simulink model "ProjectGroup5_Simulinkmodell_with_electric_motor_model"  (R2021a)
settings: Solver=FixedStepAuto  StartTime=0.0  StopTime=120  FixedStep=0.001  RelTol=1e-3
model workspace (MATLAB code in the model file):
  | g = 9.81;
  | m = 12600;
  | v = 0.7518;
  | r = 0.2323/2;
  | cd = 1.8;
  | p = 1;
  | A = 1.5;
  | 
  | Fd = 0.5*cd*p*A*v^2;
  | Fb = 1000*9.81*2;
  | E = v*g*m
  | wl = 60*v*4/r
  | Fm = m*g;
  | F = (-Fd-Fm+Fb)/4
  | 
  | T = F*r
undefined symbols (not defined in the file or in its folder): Gf, I_max, I_min, j, k, k2, ki, kp, L_m, L_m_hat, L_r, L_sig, magnitude, n_p, omega_1_N, psi_ref, R_a, R_R, R_R_hat, R_s, T_23, T_32, V_base, v_max
libraries: fl_lib x20, nesl_utility x10, CustomComponents_lib x6, pid_lib x2, sdl_lib x1, simulink x1
settings Model: Creator=simonmarheim  LastModifiedBy=michaerh
settings SolverCC: AlgebraicLoopSolver=TrustRegion
settings DebuggingCC: ArithmeticOperatorsInVariantConditions=warning
settings SFSimCC: CustomCodeUndefinedFunction=UseInterfaceOnly

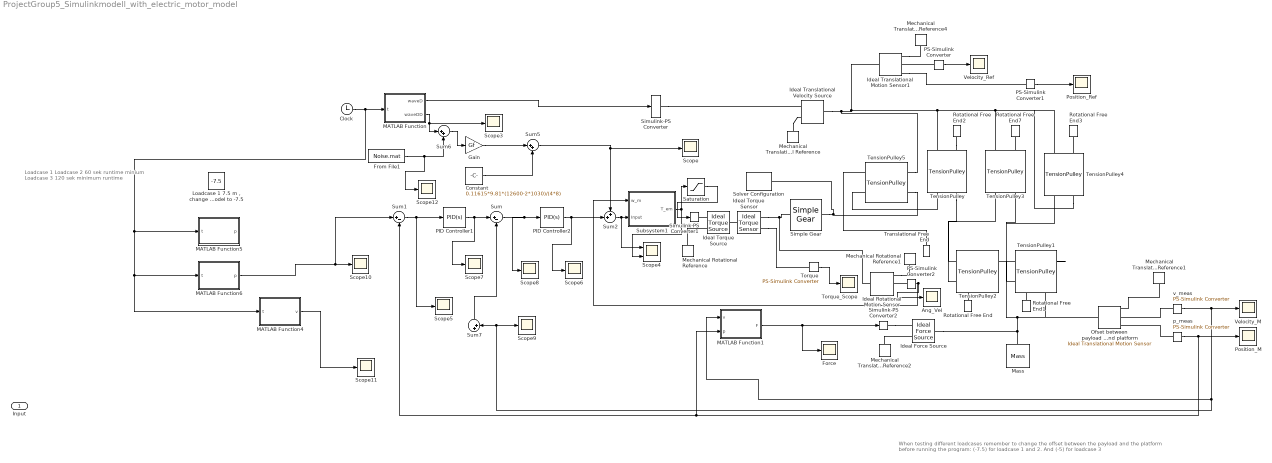
== system ProjectGroup5_Simulinkmodell_with_electric_motor_model ==
  note: Loadcase 1
      |
      | Loadcase 2
      | 60 sek runtime minium
      |
      | Loadcase 3
      | 120 sek minimum runtime
  note: When testing different loadcases remember to change the offset between the payload and the platform before running the program: (-7.5) for loadcase 1 and 2. And (-5) for loadcase 3
  Input : Inport
  Ang_Vel : Scope
  Clock : Clock
      settings: Decimation=25
  Constant : Constant  Value=0.11615*9.81*(12600-2*1030)/(4*8)
  Force : Scope
  From File1 : FromFile  FileName=Noise.mat  SampleTime=0.001
  Gain : Gain  Gain=Gf
  Ideal Force Source : fl_lib/Mechanical/Mechanical Sources/Ideal Force Source
  Ideal Rotational Motion Sensor : fl_lib/Mechanical/Mechanical Sensors/Ideal Rotational Motion Sensor  wrap_angle=simscape.enum.onoff.off  offset=0 rad
  Ideal Torque Sensor : fl_lib/Mechanical/Mechanical Sensors/Ideal Torque Sensor
  Ideal Torque Source : fl_lib/Mechanical/Mechanical Sources/Ideal Torque Source
  Ideal Translational Motion Sensor1 : fl_lib/Mechanical/Mechanical Sensors/Ideal Translational Motion Sensor  offset=0 m
  Ideal Translational Velocity Source : fl_lib/Mechanical/Mechanical Sources/Ideal Translational Velocity Source
  "Loadcase 1 7.5 m , change setpoint in model to -7.5" : Constant  Value=-7.5
  MATLAB Function : MATLAB Function  TreatAsAtomicUnit=on
  MATLAB Function1 : MATLAB Function  TreatAsAtomicUnit=on
  MATLAB Function4 : MATLAB Function  TreatAsAtomicUnit=on
  MATLAB Function5 : MATLAB Function  TreatAsAtomicUnit=on
  MATLAB Function6 : MATLAB Function  TreatAsAtomicUnit=on
  Mass : fl_lib/Mechanical/Translational Elements/Mass  mass=12600 kg  num_ports=foundation.enum.numPorts2.one  v_specify=off  v_priority=High  v=0 m/s  v_nominal_specify=off  v_nominal_unit=m/s  v_nominal_value=1  f_specify=off  f_priority=None  f=0 N  f_nominal_specify=off  f_nominal_unit=N  f_nominal_value=1
  Mechanical Rotational Reference : fl_lib/Mechanical/Rotational Elements/Mechanical Rotational Reference
  Mechanical Rotational Reference1 : fl_lib/Mechanical/Rotational Elements/Mechanical Rotational Reference
  Mechanical Translational Reference{,1..2,4} (4 alike) : fl_lib/Mechanical/Translational Elements/Mechanical Translational Reference
  Ofset between payload and platform : fl_lib/Mechanical/Mechanical Sensors/Ideal Translational Motion Sensor  offset=-5 m
  PID Controller1 : pid_lib/PID Controller  Controller=PID  Form=Parallel  TimeDomain=Continuous-time  UseExternalTs=off  SampleTime=-1  IntegratorMethod=Forward Euler  FilterMethod=Forward Euler  ControllerParametersSource=internal  P=950  I=100  D=0  UseFilter=on  N=100  TunerSelectOption=Transfer Function Based (PID Tuner App)  InitialConditionSource=internal  InitialConditionForIntegrator=0  InitialConditionForFilter=0  DifferentiatorICPrevScaledInput=0  ExternalReset=none  TrackingMode=off  Kt=1  LimitOutput=off  SatLimitsSource=internal  UpperSaturationLimit=inf  LowerSaturationLimit=-inf  LinearizeAsGain=on  AntiWindupMode=none  Kb=1  POutMin=[]  POutMax=[]  IOutMin=[]  IOutMax=[]  DOutMin=[]  DOutMax=[]  NOutMin=[]  NOutMax=[]  SumOutMin=[]  SumOutMax=[]  SaturationOutMin=[]  SaturationOutMax=[]  PParamMin=[]  PParamMax=[]  IParamMin=[]  IParamMax=[]  DParamMin=[]  DParamMax=[]  NParamMin=[]  NParamMax=[]  KbParamMin=[]  KbParamMax=[]  KtParamMin=[]  KtParamMax=[]  KbOutMin=[]  KbOutMax=[]  KtOutMin=[]  KtOutMax=[]  IntegratorOutMin=[]  IntegratorOutMax=[]  FilterOutMin=[]  FilterOutMax=[]  SumI1OutMin=[]  SumI1OutMax=[]  SumI2OutMin=[]  SumI2OutMax=[]  SumI3OutMin=[]  SumI3OutMax=[]  SumI4OutMin=[]  SumI4OutMax=[]  SumDOutMin=[]  SumDOutMax=[]  DifferentiatorOutMin=[]  DifferentiatorOutMax=[]  FilterDiffOutCoefMin=[]  FilterDiffOutCoefMax=[]  ReciprocalOutMin=[]  ReciprocalOutMax=[]  SumDenOutMin=[]  SumDenOutMax=[]  SumNumOutMin=[]  SumNumOutMax=[]  DivideOutMin=[]  DivideOutMax=[]  UdiffTsProdOutMin=[]  UdiffTsProdOutMax=[]  NTsProdOutMin=[]  NTsProdOutMax=[]  UintegralTsProdOutMin=[]  UintegralTsProdOutMax=[]  UngainTsProdOutMin=[]  UngainTsProdOutMax=[]  IntegratorContinuousStateAttributes=''  IntegratorStateMustResolveToSignalObject=off  IntegratorRTWStateStorageClass=Auto  FilterContinuousStateAttributes=''  FilterStateMustResolveToSignalObject=off  FilterRTWStateStorageClass=Auto  ParallelPVariant=InternalParameters  IdealPVariant=Disabled  IVariant=InternalParameters  DVariant=InternalParameters  IntegratorVariant=Continuous  SatVariant=Disabled  AWVariant=Passthrough  PCopyVariant=Disabled  TRVariant=Disabled  FdbkBlocksVariant=Forward  IdealPFdbkVariant=Disabled  SatFdbkVariant=Disabled  DerivativeFilterVariant=ContFilter  NVariant=InternalParameters  NCopyVariant=Disabled  FilterICVariant=InternalICsFilter  IntegratorICVariant=InternalICs  ExternalResetVariant=Disabled  TRSumVariant=Passthrough  SumFdbkVariant=Disabled  SumVariant=Sum_PID  TsampFilterVariant=InternalTs  TsampNgainVariant=Passthrough  TsampIntegralVariant=Passthrough  ExternalSaturationOutDataTypeStr=Inherit: Same as second input
  PID Controller2 : pid_lib/PID Controller  Controller=PID  Form=Parallel  TimeDomain=Continuous-time  UseExternalTs=off  SampleTime=-1  IntegratorMethod=Forward Euler  FilterMethod=Forward Euler  ControllerParametersSource=internal  P=760  I=50  D=10  UseFilter=on  N=100  TunerSelectOption=Transfer Function Based (PID Tuner App)  InitialConditionSource=internal  InitialConditionForIntegrator=0  InitialConditionForFilter=0  DifferentiatorICPrevScaledInput=0  ExternalReset=none  TrackingMode=off  Kt=1  LimitOutput=off  SatLimitsSource=internal  UpperSaturationLimit=inf  LowerSaturationLimit=-inf  LinearizeAsGain=on  AntiWindupMode=none  Kb=1  POutMin=[]  POutMax=[]  IOutMin=[]  IOutMax=[]  DOutMin=[]  DOutMax=[]  NOutMin=[]  NOutMax=[]  SumOutMin=[]  SumOutMax=[]  SaturationOutMin=[]  SaturationOutMax=[]  PParamMin=[]  PParamMax=[]  IParamMin=[]  IParamMax=[]  DParamMin=[]  DParamMax=[]  NParamMin=[]  NParamMax=[]  KbParamMin=[]  KbParamMax=[]  KtParamMin=[]  KtParamMax=[]  KbOutMin=[]  KbOutMax=[]  KtOutMin=[]  KtOutMax=[]  IntegratorOutMin=[]  IntegratorOutMax=[]  FilterOutMin=[]  FilterOutMax=[]  SumI1OutMin=[]  SumI1OutMax=[]  SumI2OutMin=[]  SumI2OutMax=[]  SumI3OutMin=[]  SumI3OutMax=[]  SumI4OutMin=[]  SumI4OutMax=[]  SumDOutMin=[]  SumDOutMax=[]  DifferentiatorOutMin=[]  DifferentiatorOutMax=[]  FilterDiffOutCoefMin=[]  FilterDiffOutCoefMax=[]  ReciprocalOutMin=[]  ReciprocalOutMax=[]  SumDenOutMin=[]  SumDenOutMax=[]  SumNumOutMin=[]  SumNumOutMax=[]  DivideOutMin=[]  DivideOutMax=[]  UdiffTsProdOutMin=[]  UdiffTsProdOutMax=[]  NTsProdOutMin=[]  NTsProdOutMax=[]  UintegralTsProdOutMin=[]  UintegralTsProdOutMax=[]  UngainTsProdOutMin=[]  UngainTsProdOutMax=[]  IntegratorContinuousStateAttributes=''  IntegratorStateMustResolveToSignalObject=off  IntegratorRTWStateStorageClass=Auto  FilterContinuousStateAttributes=''  FilterStateMustResolveToSignalObject=off  FilterRTWStateStorageClass=Auto  ParallelPVariant=InternalParameters  IdealPVariant=Disabled  IVariant=InternalParameters  DVariant=InternalParameters  IntegratorVariant=Continuous  SatVariant=Disabled  AWVariant=Passthrough  PCopyVariant=Disabled  TRVariant=Disabled  FdbkBlocksVariant=Forward  IdealPFdbkVariant=Disabled  SatFdbkVariant=Disabled  DerivativeFilterVariant=ContFilter  NVariant=InternalParameters  NCopyVariant=Disabled  FilterICVariant=InternalICsFilter  IntegratorICVariant=InternalICs  ExternalResetVariant=Disabled  TRSumVariant=Passthrough  SumFdbkVariant=Disabled  SumVariant=Sum_PID  TsampFilterVariant=InternalTs  TsampNgainVariant=Passthrough  TsampIntegralVariant=Passthrough  ExternalSaturationOutDataTypeStr=Inherit: Same as second input
  PS-Simulink Converter : nesl_utility/PS-Simulink Converter  PhysicalDomain=network_engine_domain  SubClassName=ps_output  LeftPortType=input  RightPortType=output  PseudoPeriodic=off  Frequencies=[]  Unit=inherit  AffineConversion=off
      settings: SourceProductBaseCode=PW,SS
  PS-Simulink Converter1 : nesl_utility/PS-Simulink Converter  PhysicalDomain=network_engine_domain  SubClassName=ps_output  LeftPortType=input  RightPortType=output  PseudoPeriodic=off  Frequencies=[]  Unit=inherit  AffineConversion=off
      settings: SourceProductBaseCode=PW,SS
  PS-Simulink Converter2 : nesl_utility/PS-Simulink Converter  PhysicalDomain=network_engine_domain  SubClassName=ps_output  LeftPortType=input  RightPortType=output  PseudoPeriodic=off  Frequencies=[]  Unit=inherit  AffineConversion=off
      settings: SourceProductBaseCode=PW,SS
  Position_M : Scope
  Position_Ref : Scope
  Rotational Free End{,1..3,7} (5 alike) : fl_lib/Mechanical/Rotational Elements/Rotational Free End  w_specify=off  w_priority=None  w=0 rad/s  w_nominal_specify=off  w_nominal_unit=rad/s  w_nominal_value=1
      settings: SourceProductBaseCode=SS
  Saturation : Saturate  UpperLimit=2.2*706  LowerLimit=-2.2*706
  Scope{,3,5..12} (10 alike) : Scope
  Scope4 : Scope  NumInputPorts=2
  Simple Gear : sdl_lib/Gears/Simple Gear  ratio=8  rotation_direction=sdl.enum.shaftOutputDirection.opposite  friction_model=sdl.enum.gear_efficiencies_load.off  mu_visc=[0, 0] N*m/(rad/s)  T_noload=0.1 N*m  T_nom=5 N*m  efficiency_nom=0.8  efficiency=0.8  temperature_TLU=[280, 300, 320] K  load_TLU=[1, 5, 10] N*m  efficiency_TLU=[.95, .9, .85]  efficiency_TLU2=[.85, .8, .75; .95, .9, .85; .85, .8, .7]  w_thr=0.01 rad/s  pwr_thr=0.001 W  thermal_mass=50 J/K  enable_faults=simscape.enum.onoff.off  efficiency_fault=0.05  external_fault=simscape.enum.onoff.off  temporal_fault=simscape.enum.onoff.off  fault_time=5 s  fault_angles=pi / 12 rad  report_fault=simscape.enum.assert.action.none  temperature_specify=off  temperature_priority=High  temperature=300 K  temperature_nominal_specify=off  temperature_nominal_unit=K  temperature_nominal_value=1
  Simulink-PS Converter : nesl_utility/Simulink-PS Converter  PhysicalDomain=network_engine_domain  SubClassName=ps_input  LeftPortType=input  RightPortType=output  PseudoPeriodic=off  Frequencies=[]  NoiseDistribution=none  NoiseParameters=[]  Unit=m/s  AffineConversion=off  FilteringAndDerivatives=filter  SimscapeFilterOrder=1  InputFilterTimeConstant=0.001  UdotUserProvided=0
      settings: SourceProductBaseCode=PW,SS
  Simulink-PS Converter1 : nesl_utility/Simulink-PS Converter  PhysicalDomain=network_engine_domain  SubClassName=ps_input  LeftPortType=input  RightPortType=output  PseudoPeriodic=off  Frequencies=[]  NoiseDistribution=none  NoiseParameters=[]  Unit=1  AffineConversion=off  FilteringAndDerivatives=provide  SimscapeFilterOrder=1  InputFilterTimeConstant=0.001  UdotUserProvided=0
      settings: SourceProductBaseCode=PW,SS
  Simulink-PS Converter2 : nesl_utility/Simulink-PS Converter  PhysicalDomain=network_engine_domain  SubClassName=ps_input  LeftPortType=input  RightPortType=output  PseudoPeriodic=off  Frequencies=[]  NoiseDistribution=none  NoiseParameters=[]  Unit=1  AffineConversion=off  FilteringAndDerivatives=provide  SimscapeFilterOrder=1  InputFilterTimeConstant=0.001  UdotUserProvided=0
      settings: SourceProductBaseCode=PW,SS
  Solver Configuration : nesl_utility/Solver Configuration  PhysicalDomain=network_engine_domain  SubClassName=solver  LeftPortType=input  RightPortType=generic  Tones=[]  Harmonics=[]  SimulateNoise=off  Profile=off  UseLocalSampling=off  EnableSwitchedLinearOptims=on  FrequencyDomain=off  UseCCode=off  RelTol=0.001  AbsTol=1e-06  MinStep=1e-09  ToWorkspace=off  RevertToSquareIcSolve=off  NumHomotopyIterations=100  PhasorMode=off  PhasorModeNumHarmonics=1  DoDC=off  ResidualTolerance=1e-6  UseLocalSolver=off  LocalSolverChoice=NE_BACKWARD_EULER_ADVANCER  LocalSolverSampleTime=0.001  DoFixedCost=off  MaxNonlinIter=100  MaxModeIter=10  ComputeImpulses=off  ImpulseIterations=2  LinearAlgebra=auto  EquationFormulation=NE_TIME_EF  DelaysMemoryBudget=1024  AutomaticFiltering=on  FilteringTimeConstant=0.001  PartitionStorageMethod=AS_NEEDED  PartitionMemoryBudget=1024  PartitionMethod=ROBUST
      settings: SourceProductBaseCode=PW,SS
  Subsystem1 : Subsystem
  Sum : Sum  Inputs=|+-
  Sum1 : Sum  Inputs=|+-
  Sum2 : Sum  Inputs=++|
  Sum5 : Sum  Inputs=|++
  Sum6 : Sum  Inputs=|++
  Sum7 : Sum  Inputs=|++
  TensionPulley{,1..4} (5 alike) : CustomComponents_lib/TensionPulley  radius=0.1 m  b_damp=0.001 N*m*s/rad  inertia=0.01 kg*m^2  mass=1 kg  mu_s=1  f_A_specify=off  f_A_priority=None  f_A=0 N  f_A_nominal_specify=off  f_A_nominal_unit=N  f_A_nominal_value=1  f_B_specify=off  f_B_priority=None  f_B=0 N  f_B_nominal_specify=off  f_B_nominal_unit=N  f_B_nominal_value=1  f_C_specify=off  f_C_priority=None  f_C=0 N  f_C_nominal_specify=off  f_C_nominal_unit=N  f_C_nominal_value=1  tau_specify=off  tau_priority=None  tau=0 N*m  tau_nominal_specify=off  tau_nominal_unit=N*m  tau_nominal_value=1  w_specify=off  w_priority=None  w=0 rad/s  w_nominal_specify=off  w_nominal_unit=rad/s  w_nominal_value=1  v_specify=off  v_priority=None  v=0 m/s  v_nominal_specify=off  v_nominal_unit=m/s  v_nominal_value=1
      settings: InternalSimscapePortConfiguration="{\"Bottom\":[],\"Left\":[{\"id\":\"C\",\"label\":\"C\",\"type\":\"foundation.mechanical.translational.translational\"},{\"id\":\"S\",\"label\":\"S\",\"type\":\"foundation.mechanical.rotational.rotational\"}],\"Right\":[{\"id\":\"A\",\"label\":\"A\",\"type\":\"foundation.mechanical.translational.translational\"},{\"id\":\"B\",\"label\":\"B\",\"type\":\"foundation.mechanical.translational.translational\"}],\"Top\":[]}"
  TensionPulley5 : CustomComponents_lib/TensionPulley  radius=11.615 cm  b_damp=0.001 N*m/(rad/s)  inertia=1 kg*m^2  mass=1 kg  mu_s=1  f_A_specify=off  f_A_priority=None  f_A=0 N  f_A_nominal_specify=off  f_A_nominal_unit=N  f_A_nominal_value=1  f_B_specify=off  f_B_priority=None  f_B=0 N  f_B_nominal_specify=off  f_B_nominal_unit=N  f_B_nominal_value=1  f_C_specify=off  f_C_priority=None  f_C=0 N  f_C_nominal_specify=off  f_C_nominal_unit=N  f_C_nominal_value=1  tau_specify=off  tau_priority=None  tau=0 N*m  tau_nominal_specify=off  tau_nominal_unit=N*m  tau_nominal_value=1  w_specify=off  w_priority=None  w=0 rad/s  w_nominal_specify=off  w_nominal_unit=rad/s  w_nominal_value=1  v_specify=off  v_priority=None  v=0 m/s  v_nominal_specify=off  v_nominal_unit=m/s  v_nominal_value=1
      settings: InternalSimscapePortConfiguration="{\"Bottom\":[],\"Left\":[{\"id\":\"C\",\"label\":\"C\",\"type\":\"foundation.mechanical.translational.translational\"},{\"id\":\"S\",\"label\":\"S\",\"type\":\"foundation.mechanical.rotational.rotational\"}],\"Right\":[{\"id\":\"A\",\"label\":\"A\",\"type\":\"foundation.mechanical.translational.translational\"},{\"id\":\"B\",\"label\":\"B\",\"type\":\"foundation.mechanical.translational.translational\"}],\"Top\":[]}"
  Torque : nesl_utility/PS-Simulink Converter  PhysicalDomain=network_engine_domain  SubClassName=ps_output  LeftPortType=input  RightPortType=output  PseudoPeriodic=off  Frequencies=[]  Unit=inherit  AffineConversion=off
      settings: SourceProductBaseCode=PW,SS
  Torque_Scope : Scope
  Translational Free End : fl_lib/Mechanical/Translational Elements/Translational Free End  v_specify=off  v_priority=None  v=0 m/s  v_nominal_specify=off  v_nominal_unit=m/s  v_nominal_value=1
      settings: SourceProductBaseCode=SS  InternalSimscapePortConfiguration="{\"Bottom\":[],\"Left\":[{\"id\":\"V\",\"label\":\"\",\"type\":\"foundation.mechanical.translational.translational\"}],\"Right\":[],\"Top\":[]}"
  Velocity_M : Scope
  Velocity_Ref : Scope
  p_meas : nesl_utility/PS-Simulink Converter  PhysicalDomain=network_engine_domain  SubClassName=ps_output  LeftPortType=input  RightPortType=output  PseudoPeriodic=off  Frequencies=[]  Unit=inherit  AffineConversion=off
      settings: SourceProductBaseCode=PW,SS
  v_meas : nesl_utility/PS-Simulink Converter  PhysicalDomain=network_engine_domain  SubClassName=ps_output  LeftPortType=input  RightPortType=output  PseudoPeriodic=off  Frequencies=[]  Unit=inherit  AffineConversion=off
      settings: SourceProductBaseCode=PW,SS
  wires:
  Clock/1 -> MATLAB Function5/1(t), MATLAB Function6/1(t), MATLAB Function4/1(t), MATLAB Function/1(t)
  p_meas/1 -> Position_M/1, MATLAB Function1/2(p), Sum1/2
  Sum1/1 -> Scope5/1, PID Controller1/1
  Torque/1 -> Torque_Scope/1
  PS-Simulink Converter/1 -> Velocity_Ref/1
  PS-Simulink Converter1/1 -> Position_Ref/1
  Sum/1 -> Scope8/1, PID Controller2/1
  PS-Simulink Converter2/1 -> Subsystem1/1(w_m), Ang_Vel/1
  MATLAB Function1/1(F) -> Force/1, Simulink-PS Converter2/1
  MATLAB Function/1(waveD) -> Simulink-PS Converter/1
  Gain/1 -> Sum5/1
  Constant/1 -> Sum5/2
  Sum5/1 -> Sum2/1, Scope/1
  PID Controller1/1 -> Scope7/1, Sum/1
  From File1/1 -> Scope12/1, Sum6/2
  MATLAB Function/2(waveDD) -> Scope3/1, Sum6/1
  Sum6/1 -> Gain/1
  Sum2/1 -> Subsystem1/2(Input), Scope4/1
  Subsystem1/1(T_em) -> Scope4/2, Saturation/1
  PID Controller2/1 -> Scope6/1, Sum2/2
  v_meas/1 -> Sum7/2, Scope9/1, MATLAB Function1/1(v), Velocity_M/1
  Sum7/1 -> Sum/2
  MATLAB Function4/1(v) -> Scope11/1
  Saturation/1 -> Simulink-PS Converter1/1
  MATLAB Function6/1(p) -> Sum1/1, Scope10/1
  connections:
  TensionPulley5/LConn2 -- Solver Configuration/RConn1 -- Simple Gear/RConn1
  TensionPulley2/LConn1 -- TensionPulley1/LConn1 -- Ofset between payload and platform/LConn1 -- Ideal Force Source/LConn1 -- Mass/LConn1
  Rotational Free End/LConn1 -- TensionPulley2/LConn2
  Ofset between payload and platform/RConn1 -- Mechanical Translational Reference1/LConn1
  TensionPulley4/LConn2 -- Rotational Free End3/LConn1
  TensionPulley3/LConn2 -- Rotational Free End7/LConn1
  TensionPulley2/RConn1 -- TensionPulley3/RConn1
  TensionPulley1/RConn1 -- TensionPulley4/RConn1
  TensionPulley/RConn2 -- TensionPulley2/RConn2
  Ideal Torque Source/RConn1 -- Simulink-PS Converter1/RConn1
  v_meas/LConn1 -- Ofset between payload and platform/RConn2
  Rotational Free End2/LConn1 -- TensionPulley/LConn2
  TensionPulley1/RConn2 -- TensionPulley3/RConn2
  Rotational Free End1/LConn1 -- TensionPulley1/LConn2
  Ideal Torque Source/RConn2 -- Mechanical Rotational Reference/LConn1
  Simulink-PS Converter2/RConn1 -- Ideal Force Source/RConn1
  Mechanical Translational Reference2/LConn1 -- Ideal Force Source/RConn2
  p_meas/LConn1 -- Ofset between payload and platform/RConn3
  Simulink-PS Converter/RConn1 -- Ideal Translational Velocity Source/RConn1
  PS-Simulink Converter/LConn1 -- Ideal Translational Motion Sensor1/RConn2
  Ideal Translational Motion Sensor1/RConn1 -- Mechanical Translational Reference4/LConn1
  Ideal Translational Velocity Source/LConn1 -- TensionPulley5/LConn1 -- TensionPulley3/LConn1 -- TensionPulley4/RConn2 -- TensionPulley4/LConn1 -- TensionPulley/LConn1 -- Ideal Translational Motion Sensor1/LConn1
  Mechanical Translational Reference/LConn1 -- Ideal Translational Velocity Source/RConn2
  TensionPulley5/RConn1 -- Translational Free End/LConn1
  TensionPulley5/RConn2 -- TensionPulley/RConn1
  Ideal Translational Motion Sensor1/RConn3 -- PS-Simulink Converter1/LConn1
  Ideal Torque Sensor/LConn1 -- Ideal Torque Source/LConn1
  Ideal Torque Sensor/RConn2 -- Torque/LConn1
  Ideal Torque Sensor/RConn1 -- Ideal Rotational Motion Sensor/LConn1 -- Simple Gear/LConn1
  PS-Simulink Converter2/LConn1 -- Ideal Rotational Motion Sensor/RConn2
  Ideal Rotational Motion Sensor/RConn1 -- Mechanical Rotational Reference1/LConn1

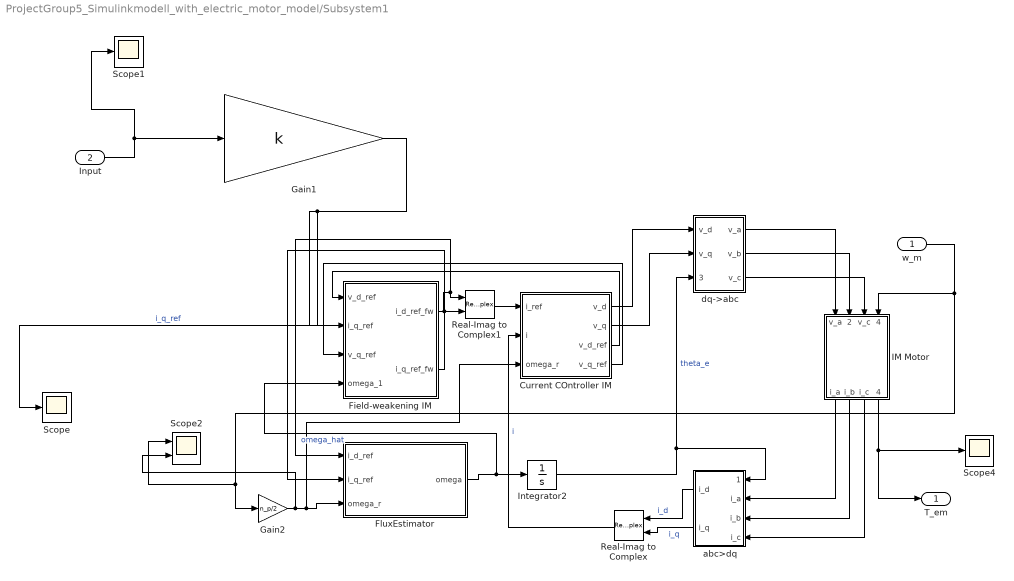
== system ProjectGroup5_Simulinkmodell_with_electric_motor_model/Subsystem1 ==
  w_m : Inport
  Input : Inport  Port=2
  Current COntroller IM : Subsystem
  Field-weakening IM : Subsystem
  FluxEstimator : Subsystem
  Gain1 : Gain  Gain=k
  Gain2 : Gain  Gain=n_p/2
  IM Motor : Subsystem
  Integrator2 : Integrator
  Real-Imag to Complex : RealImagToComplex
  Real-Imag to Complex1 : RealImagToComplex
  Scope : Scope
  Scope1 : Scope
  Scope2 : Scope  NumInputPorts=2
  Scope4 : Scope
  abc>dq : Subsystem
  dq->abc : Subsystem
  T_em : Outport
  wires:
  Current COntroller IM/4(v_q_ref) -> Field-weakening IM/3(v_q_ref)
  Input/1 -> Gain1/1, Scope1/1
  abc>dq/1(i_d) -> Real-Imag to Complex/1  "i_d"
  IM Motor/4(T_em) -> T_em/1, Scope4/1
  FluxEstimator/1(omega) -> Field-weakening IM/4(omega_1), Integrator2/1  "omega_hat"
  dq->abc/2(v_b) -> IM Motor/2(v_b)
  dq->abc/1(v_a) -> IM Motor/1(v_a)
  Gain2/1 -> Scope2/2, Current COntroller IM/3(omega_r), FluxEstimator/3(omega_r)
  Field-weakening IM/2(i_q_ref_fw) -> FluxEstimator/2(i_q_ref), Real-Imag to Complex1/2
  Current COntroller IM/2(v_q) -> dq->abc/2(v_q)
  w_m/1 -> Gain2/1, Scope2/1, IM Motor/4(w_m)
  Real-Imag to Complex1/1 -> Current COntroller IM/1(i_ref)
  Field-weakening IM/1(i_d_ref_fw) -> Real-Imag to Complex1/1, FluxEstimator/1(i_d_ref)
  Integrator2/1 -> dq->abc/3(theta_e), abc>dq/1(theta_e)  "theta_e"
  IM Motor/3(i_c) -> abc>dq/4(i_c)
  Real-Imag to Complex/1 -> Current COntroller IM/2(i)  "i"
  IM Motor/1(i_a) -> abc>dq/2(i_a)
  Current COntroller IM/3(v_d_ref) -> Field-weakening IM/1(v_d_ref)
  IM Motor/2(i_b) -> abc>dq/3(i_b)
  abc>dq/2(i_q) -> Real-Imag to Complex/2  "i_q"
  dq->abc/3(v_c) -> IM Motor/3(v_c)
  Current COntroller IM/1(v_d) -> dq->abc/1(v_d)
  Gain1/1 -> Scope/1, Field-weakening IM/2(i_q_ref)  "i_q_ref"

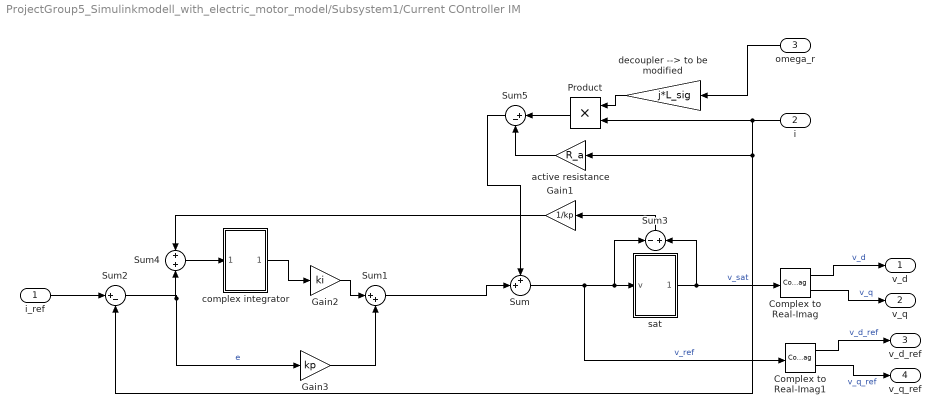
== system ProjectGroup5_Simulinkmodell_with_electric_motor_model/Subsystem1/Current COntroller IM ==
  i_ref : Inport
  i : Inport  Port=2
  omega_r : Inport  Port=3
  Complex to Real-Imag : ComplexToRealImag
  Complex to Real-Imag1 : ComplexToRealImag
  Gain1 : Gain  Gain=1/kp
  Gain2 : Gain  Gain=ki
  Gain3 : Gain  Gain=kp
  Product : Product
  Sum : Sum  Inputs=++|
  Sum1 : Sum  Inputs=|++
  Sum2 : Sum  Inputs=|+-
  Sum3 : Sum  Inputs=-|+
  Sum4 : Sum
  Sum5 : Sum  Inputs=|+-
  active resistance : Gain  Gain=R_a
  complex integrator : Subsystem
  "decoupler --> to be modified " : Gain  Gain=j*L_sig
  sat : Subsystem
  v_d : Outport
  v_q : Outport  Port=2
  v_d_ref : Outport  Port=3
  v_q_ref : Outport  Port=4
  wires:
  Complex to Real-Imag/2 -> v_q/1  "v_q"
  Complex to Real-Imag/1 -> v_d/1  "v_d"
  "decoupler --> to be modified "/1 -> Product/1
  Sum5/1 -> Sum/1
  complex integrator/1(Out1) -> Gain2/1
  Product/1 -> Sum5/1
  active resistance/1 -> Sum5/2
  omega_r/1 -> "decoupler --> to be modified "/1
  Sum2/1 -> Sum4/2, Gain3/1  "e"
  i_ref/1 -> Sum2/1
  i/1 -> Sum2/2, active resistance/1, Product/2
  Gain2/1 -> Sum1/1
  Gain3/1 -> Sum1/2
  Sum1/1 -> Sum/2
  Sum3/1 -> Gain1/1
  sat/1(v_sat) -> Complex to Real-Imag/1, Sum3/2  "v_sat"
  Sum4/1 -> complex integrator/1(In1)
  Gain1/1 -> Sum4/1
  Sum/1 -> Complex to Real-Imag1/1, Sum3/1, sat/1(v)  "v_ref"
  Complex to Real-Imag1/1 -> v_d_ref/1  "v_d_ref"
  Complex to Real-Imag1/2 -> v_q_ref/1  "v_q_ref"

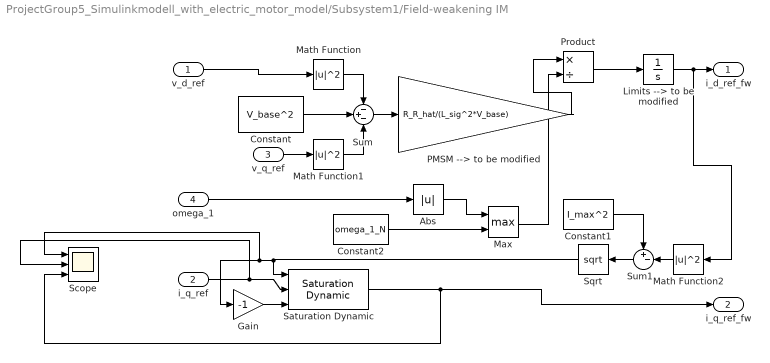
== system ProjectGroup5_Simulinkmodell_with_electric_motor_model/Subsystem1/Field-weakening IM ==
  v_d_ref : Inport
  i_q_ref : Inport  Port=2
  v_q_ref : Inport  Port=3
  omega_1 : Inport  Port=4
  Abs : Abs
  Constant : Constant  Value=V_base^2
  Constant1 : Constant  Value=I_max^2
  Constant2 : Constant  Value=omega_1_N
  Gain : Gain  Gain=-1
  Limits --> to be modified : Integrator  InitialCondition=I_min  LimitOutput=on  UpperSaturationLimit=psi_ref/L_m_hat  LowerSaturationLimit=I_min
  Math Function : Math  Operator=magnitude^2  SaturateOnIntegerOverflow=on
  Math Function1 : Math  Operator=magnitude^2  SaturateOnIntegerOverflow=on
  Math Function2 : Math  Operator=magnitude^2  SaturateOnIntegerOverflow=on
  Max : MinMax  Function=max  Inputs=2
  PMSM --> to be modified : Gain  Gain=R_R_hat/(L_sig^2*V_base)
  Product : Product  Inputs=*/
  Saturation Dynamic : simulink/Discontinuities/Saturation Dynamic  OutMin=[]  OutMax=[]  OutDataTypeStr=Inherit: Same as second input  OutDataType=fixdt(1, 16)  OutScaling=2^-10  DoSatur=off
  Scope : Scope  NumInputPorts=3
  Sqrt : Sqrt  SaturateOnIntegerOverflow=on
  Sum : Sum  Inputs=-+-
  Sum1 : Sum  Inputs=+-|
  i_d_ref_fw : Outport
  i_q_ref_fw : Outport  Port=2
  wires:
  i_q_ref/1 -> Scope/2, Saturation Dynamic/2
  v_d_ref/1 -> Math Function/1
  v_q_ref/1 -> Math Function1/1
  Constant/1 -> Sum/2
  Math Function/1 -> Sum/1
  Math Function1/1 -> Sum/3
  Sum/1 -> PMSM --> to be modified/1
  PMSM --> to be modified/1 -> Product/1
  omega_1/1 -> Abs/1
  Abs/1 -> Max/1
  Max/1 -> Product/2
  Product/1 -> Limits --> to be modified/1
  Limits --> to be modified/1 -> Math Function2/1, i_d_ref_fw/1
  Math Function2/1 -> Sum1/2
  Constant1/1 -> Sum1/1
  Sum1/1 -> Sqrt/1
  Sqrt/1 -> Scope/1, Gain/1, Saturation Dynamic/1
  Gain/1 -> Saturation Dynamic/3
  Saturation Dynamic/1 -> Scope/3, i_q_ref_fw/1
  Constant2/1 -> Max/2

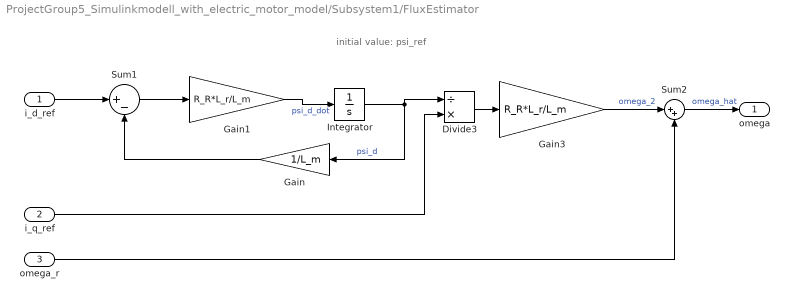
== system ProjectGroup5_Simulinkmodell_with_electric_motor_model/Subsystem1/FluxEstimator ==
  note: initial value: psi_ref
  i_d_ref : Inport
  i_q_ref : Inport  Port=2
  omega_r : Inport  Port=3
  Divide3 : Product  Inputs=/*
  Gain : Gain  Gain=1/L_m
  Gain1 : Gain  Gain=R_R*L_r/L_m
  Gain3 : Gain  Gain=R_R*L_r/L_m
  Integrator : Integrator  InitialCondition=psi_ref
  Sum1 : Sum  Inputs=|+-
  Sum2 : Sum  Inputs=|++
  omega : Outport  VectorParamsAs1DForOutWhenUnconnected=off
  wires:
  Gain1/1 -> Integrator/1  "psi_d_dot"
  Gain/1 -> Sum1/2
  Integrator/1 -> Divide3/1, Gain/1  "psi_d"
  i_d_ref/1 -> Sum1/1
  Sum1/1 -> Gain1/1
  i_q_ref/1 -> Divide3/2
  Divide3/1 -> Gain3/1
  Gain3/1 -> Sum2/1  "omega_2"
  Sum2/1 -> omega/1  "omega_hat"
  omega_r/1 -> Sum2/2

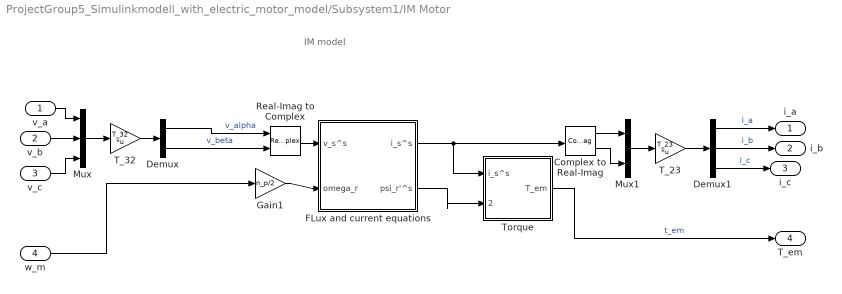
== system ProjectGroup5_Simulinkmodell_with_electric_motor_model/Subsystem1/IM Motor ==
  note: IM model
  v_a : Inport
  v_b : Inport  Port=2
  v_c : Inport  Port=3
  w_m : Inport  Port=4
  Complex to Real-Imag : ComplexToRealImag
  Demux : Demux  Outputs=2
  Demux1 : Demux  Outputs=3
  FLux and current equations : Subsystem
  Gain1 : Gain  Gain=n_p/2
  Mux : Mux  Inputs=3
  Mux1 : Mux  Inputs=2
  Real-Imag to Complex : RealImagToComplex
  T_23 : Gain  Gain=T_23  Multiplication=Matrix(K*u)
  T_32 : Gain  Gain=T_32  Multiplication=Matrix(K*u)
  Torque : Subsystem
  i_a : Outport
  i_b : Outport  Port=2
  i_c : Outport  Port=3
  T_em : Outport  Port=4
  wires:
  Demux1/1 -> i_a/1  "i_a"
  v_b/1 -> Mux/2
  Torque/1(T_em) -> T_em/1  "t_em"
  Mux/1 -> T_32/1
  v_a/1 -> Mux/1
  Demux/1 -> Real-Imag to Complex/1  "v_alpha"
  FLux and current equations/1(i_s^s) -> Complex to Real-Imag/1, Torque/1(i_s^s)
  Complex to Real-Imag/2 -> Mux1/2
  FLux and current equations/2(psi_r'^s) -> Torque/2(psi_r^s)
  Real-Imag to Complex/1 -> FLux and current equations/1(v_s^s)
  v_c/1 -> Mux/3
  Demux1/2 -> i_b/1  "i_b"
  Demux/2 -> Real-Imag to Complex/2  "v_beta"
  Mux1/1 -> T_23/1
  T_32/1 -> Demux/1
  Complex to Real-Imag/1 -> Mux1/1
  Demux1/3 -> i_c/1  "i_c"
  Gain1/1 -> FLux and current equations/2(omega_r)
  T_23/1 -> Demux1/1
  w_m/1 -> Gain1/1

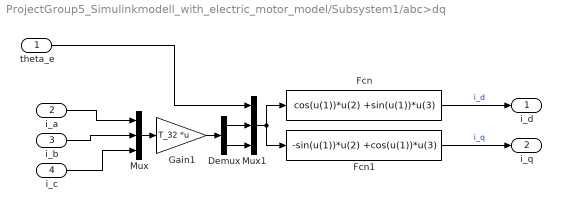
== system ProjectGroup5_Simulinkmodell_with_electric_motor_model/Subsystem1/abc>dq ==
  theta_e : Inport
  i_a : Inport  Port=2
  i_b : Inport  Port=3
  i_c : Inport  Port=4
  Demux : Demux  Outputs=2
  Fcn : Fcn  Expr=cos(u(1))*u(2) +sin(u(1))*u(3)
  Fcn1 : Fcn  Expr=-sin(u(1))*u(2) +cos(u(1))*u(3)
  Gain1 : Gain  Gain=T_32  Multiplication=Matrix(K*u)
  Mux : Mux  Inputs=3
  Mux1 : Mux  Inputs=3
  i_d : Outport  VectorParamsAs1DForOutWhenUnconnected=off
  i_q : Outport  Port=2  VectorParamsAs1DForOutWhenUnconnected=off
  wires:
  i_a/1 -> Mux/1
  Demux/1 -> Mux1/2
  Fcn1/1 -> i_q/1  "i_q"
  Demux/2 -> Mux1/3
  theta_e/1 -> Mux1/1
  Mux1/1 -> Fcn1/1, Fcn/1
  Gain1/1 -> Demux/1
  i_b/1 -> Mux/2
  Fcn/1 -> i_d/1  "i_d"
  i_c/1 -> Mux/3
  Mux/1 -> Gain1/1

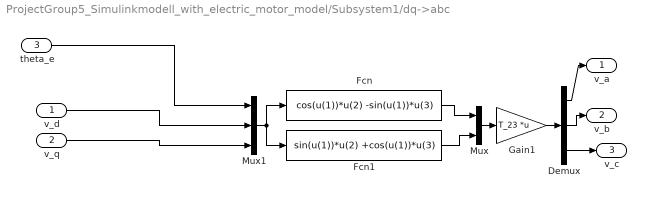
== system ProjectGroup5_Simulinkmodell_with_electric_motor_model/Subsystem1/dq->abc ==
  v_d : Inport
  v_q : Inport  Port=2
  theta_e : Inport  Port=3
  Demux : Demux  Outputs=3
  Fcn : Fcn  Expr=cos(u(1))*u(2) -sin(u(1))*u(3)
  Fcn1 : Fcn  Expr=sin(u(1))*u(2) +cos(u(1))*u(3)
  Gain1 : Gain  Gain=T_23  Multiplication=Matrix(K*u)
  Mux : Mux  Inputs=2
  Mux1 : Mux  Inputs=3
  v_a : Outport  VectorParamsAs1DForOutWhenUnconnected=off
  v_b : Outport  Port=2  VectorParamsAs1DForOutWhenUnconnected=off
  v_c : Outport  Port=3  VectorParamsAs1DForOutWhenUnconnected=off
  wires:
  v_d/1 -> Mux1/2
  v_q/1 -> Mux1/3
  theta_e/1 -> Mux1/1
  Mux1/1 -> Fcn1/1, Fcn/1
  Fcn/1 -> Mux/1
  Fcn1/1 -> Mux/2
  Mux/1 -> Gain1/1
  Gain1/1 -> Demux/1
  Demux/1 -> v_a/1
  Demux/3 -> v_c/1
  Demux/2 -> v_b/1

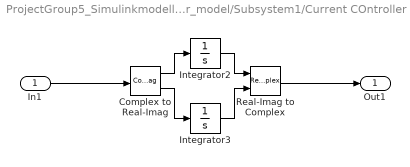
== system ProjectGroup5_Simulinkmodell_with_electric_motor_model/Subsystem1/Current COntroller IM/complex integrator ==
  In1 : Inport
  Complex to Real-Imag : ComplexToRealImag
  Integrator2 : Integrator
  Integrator3 : Integrator
  Real-Imag to Complex : RealImagToComplex
  Out1 : Outport  VectorParamsAs1DForOutWhenUnconnected=off
  wires:
  In1/1 -> Complex to Real-Imag/1
  Integrator2/1 -> Real-Imag to Complex/1
  Complex to Real-Imag/2 -> Integrator3/1
  Complex to Real-Imag/1 -> Integrator2/1
  Real-Imag to Complex/1 -> Out1/1
  Integrator3/1 -> Real-Imag to Complex/2

== system ProjectGroup5_Simulinkmodell_with_electric_motor_model/Subsystem1/Current COntroller IM/sat ==
  v : Inport
  Complex to Magnitude-Angle : ComplexToMagnitudeAngle
  Magnitude-Angle to Complex : MagnitudeAngleToComplex
  Saturation : Saturate  UpperLimit=v_max  LowerLimit=-v_max
  v_sat : Outport  VectorParamsAs1DForOutWhenUnconnected=off
  wires:
  v/1 -> Complex to Magnitude-Angle/1
  Magnitude-Angle to Complex/1 -> v_sat/1  "v_sat"
  Complex to Magnitude-Angle/1 -> Saturation/1
  Saturation/1 -> Magnitude-Angle to Complex/1
  Complex to Magnitude-Angle/2 -> Magnitude-Angle to Complex/2

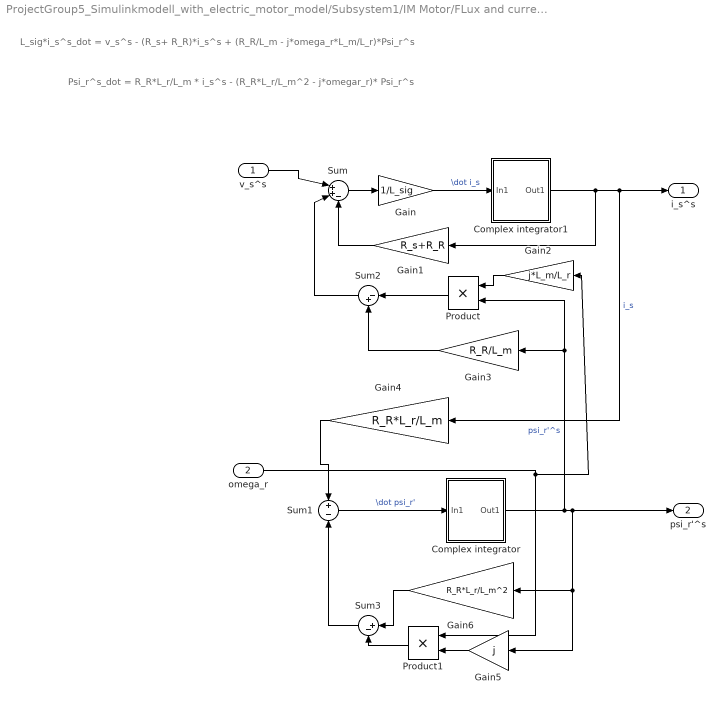
== system ProjectGroup5_Simulinkmodell_with_electric_motor_model/Subsystem1/IM Motor/FLux and current equations ==
  note: Psi_r^s_dot = R_R*L_r/L_m * i_s^s - (R_R*L_r/L_m^2 - j*omegar_r)* Psi_r^s
  note: L_sig*i_s^s_dot = v_s^s - (R_s+ R_R)*i_s^s + (R_R/L_m - j*omega_r*L_m/L_r)*Psi_r^s
  v_s^s : Inport
  omega_r : Inport  Port=2
  Complex integrator : Subsystem
  Complex integrator1 : Subsystem
  Gain : Gain  Gain=1/L_sig
  Gain1 : Gain  Gain=R_s+R_R
  Gain2 : Gain  Gain=j*L_m/L_r
  Gain3 : Gain  Gain=R_R/L_m
  Gain4 : Gain  Gain=R_R*L_r/L_m
  Gain5 : Gain  Gain=j
  Gain6 : Gain  Gain=R_R*L_r/L_m^2
  Product : Product
  Product1 : Product
  Sum : Sum  Inputs=|++-
  Sum1 : Sum  Inputs=+|-
  Sum2 : Sum  Inputs=|-+
  Sum3 : Sum  Inputs=|+-
  i_s^s : Outport
  psi_r'^s : Outport  Port=2
  wires:
  v_s^s/1 -> Sum/1
  Sum2/1 -> Sum/2
  Gain1/1 -> Sum/3
  Sum3/1 -> Sum1/2
  Gain4/1 -> Sum1/1
  Gain5/1 -> Product1/2
  Product1/1 -> Sum3/2
  Complex integrator1/1(Out1) -> i_s^s/1, Gain4/1, Gain1/1  "i_s"
  Gain2/1 -> Product/1
  omega_r/1 -> Product1/1, Gain2/1
  Gain/1 -> Complex integrator1/1(In1)  "\\dot i_s"
  Complex integrator/1(Out1) -> Gain3/1, Product/2, psi_r'^s/1, Gain6/1, Gain5/1  "psi_r'^s"
  Gain3/1 -> Sum2/2
  Sum1/1 -> Complex integrator/1(In1)  "\\dot psi_r'"
  Sum/1 -> Gain/1
  Product/1 -> Sum2/1
  Gain6/1 -> Sum3/1

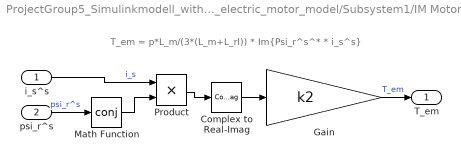
== system ProjectGroup5_Simulinkmodell_with_electric_motor_model/Subsystem1/IM Motor/Torque ==
  note: T_em = p*L_m/(3*(L_m+L_rl)) * Im{Psi_r^s^* * i_s^s}
  i_s^s : Inport
  psi_r^s : Inport  Port=2
  Complex to Real-Imag : ComplexToRealImag  Output=Imag
  Gain : Gain  Gain=k2
  Math Function : Math  Operator=conj  SignedPower=on  SaturateOnIntegerOverflow=on
  Product : Product
  T_em : Outport  VectorParamsAs1DForOutWhenUnconnected=off
  wires:
  Product/1 -> Complex to Real-Imag/1
  Math Function/1 -> Product/2
  Complex to Real-Imag/1 -> Gain/1
  Gain/1 -> T_em/1  "T_em"
  i_s^s/1 -> Product/1  "i_s"
  psi_r^s/1 -> Math Function/1  "psi_r^s"

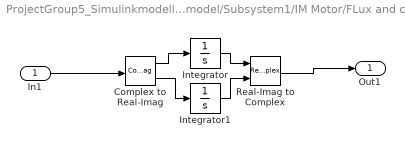
== system ProjectGroup5_Simulinkmodell_with_electric_motor_model/Subsystem1/IM Motor/FLux and current equations/Complex integrator ==
  In1 : Inport
  Complex to Real-Imag : ComplexToRealImag
  Integrator : Integrator  InitialCondition=psi_ref
  Integrator1 : Integrator
  Real-Imag to Complex : RealImagToComplex
  Out1 : Outport  VectorParamsAs1DForOutWhenUnconnected=off
  wires:
  Integrator/1 -> Real-Imag to Complex/1
  Complex to Real-Imag/1 -> Integrator/1
  Real-Imag to Complex/1 -> Out1/1
  Complex to Real-Imag/2 -> Integrator1/1
  Integrator1/1 -> Real-Imag to Complex/2
  In1/1 -> Complex to Real-Imag/1

== system ProjectGroup5_Simulinkmodell_with_electric_motor_model/Subsystem1/IM Motor/FLux and current equations/Complex integrator1 ==
  In1 : Inport
  Complex to Real-Imag : ComplexToRealImag
  Integrator : Integrator
  Integrator1 : Integrator
  Real-Imag to Complex : RealImagToComplex
  Out1 : Outport  VectorParamsAs1DForOutWhenUnconnected=off
  wires:
  Integrator/1 -> Real-Imag to Complex/1
  Complex to Real-Imag/1 -> Integrator/1
  Real-Imag to Complex/1 -> Out1/1
  Complex to Real-Imag/2 -> Integrator1/1
  Integrator1/1 -> Real-Imag to Complex/2
  In1/1 -> Complex to Real-Imag/1

== matlab function ProjectGroup5_Simulinkmodell_with_electric_motor_model/MATLAB Function1 ==
  data: F output; v input; p input
 function F   = Forces(v, p)

%Constants
g = 9.81;
m = 12600;
cd = 1.8;
rho = 1030;
A = 1.5;
V = 2;
k = 1.8E6; %N/m
b = 6.5E5; %N*s/m^1.5


%Assigning inputs
if p > -7.5
    x = 0;
    xDot = 0;
else
    x = -p - 7.5;
    xDot = -v;
end


%Calculating forces
% F_sb = k * x + b * xDot * sqrt(x); %uncomment for seabedforce
F_d = 0.5 * cd * rho * A * sign(-v) * v^2;
G = - g * m + V * rho * g;

 F = F_d + G; %+ F_sb; %uncomment for seabedforce

end

== matlab function ProjectGroup5_Simulinkmodell_with_electric_motor_model/MATLAB Function ==
  settings: updateMethod=DISCRETE
  data: t input; waveD output; waveDD output
function [waveD, waveDD]    = Wave_generation_script(t)
%Wave generation script generates stochastic waves
% Hs is the significant wave height [m]
% T is the mean period [s]
% t_end is the end time [s]
% t is the time [s]
% wave is sea surface elevation [m]
%% Input parameters
wave = 0; %[m]
w = linspace(0.1,2.0,20); % frequency range
delta_w = w(2) - w(1);
T = 10;
t_end = 60;
Hs = 1.7;

%% PM spectrum ( freq . domain )
w1 = (2 * pi) / T;
A = 0.11 * (Hs^2) * (w1^4);
B = 0.44 * (w1^4);
S = (A./w.^5) .* exp(-(B./w.^4));

%% Wave amplitude ( time domain )
%& sfr = 25; % sampling frequency (Hz) (higher freq −> higher resolution)
%t = [0: 1/sfr: t_end] ; % time vector
%phi_test = rng ;
phi = 2 * pi * ( rand(1,length(w)) - 0.5); % random phase of ith frequency [rad]
rng(0) ;
A_wave = sqrt(2*S.*delta_w) ; % amplitude of each sine wave. wave = [ ]

for i = 1 : 25*60
    wave = sum(A_wave.*cos(w*t + phi)); % [m] sea surface elevation
    waveD = sum(-A_wave.*sin(w*t + phi).*w); % [m/s] sea surface velocity
    waveDD = sum(-A_wave.*cos(w*t + phi).*w.*w); % [m/s^2] sea surface acceleration
    
%     Y(i) = wave;
%     Yd(i) = waveD;
%     Ydd(i) = waveDD;
end

end

== matlab function ProjectGroup5_Simulinkmodell_with_electric_motor_model/MATLAB Function6 ==
  data: t input; p output
function p = fcn(t)

deltas = 5; % m
T = 120; %s
tr = 5; 

v0 = deltas/(T-tr);

    if t<=tr
        p = v0/(2*tr)*t^2 - 5;
    elseif t<=T-tr
        p = v0*tr/2 + v0*(t-tr)-5;
    elseif t<=T
       p= v0/tr*(T*t-0.5*t^2)+deltas-v0*T^2/(2*tr)-5;
    else
       p = 0;
    end
        
        
        
end

== matlab function ProjectGroup5_Simulinkmodell_with_electric_motor_model/MATLAB Function4 ==
  data: t input; v output
function v = fcn(t)

deltas = 2.5; % m
T = 60; %s
tr = 5; 
v0 = deltas/(T-tr);

    if t<=tr
        v = v0*t/tr;
    elseif t<=(T-tr)
        v = v0;
    elseif t<=(T)
        v = v0*(T-t)/tr;
    else
        v = 0;
    end
        
        
        
end

== matlab function ProjectGroup5_Simulinkmodell_with_electric_motor_model/MATLAB Function5 ==
  data: t input; p output
function p = fcn(t)

deltas = 2.5; % m
T = 60; %s
tr = 5; 

v0 = deltas/(T-tr);

    if t<=tr
        p = v0/(2*tr)*t^2 - 7.5;
    elseif t<=T-tr
        p = v0*tr/2 + v0*(t-tr)-7.5;
    elseif t<=T
       p= v0/tr*(T*t-0.5*t^2)+deltas-v0*T^2/(2*tr)-7.5;
    else
       p = -5;
    end
        
        
        
end
